simulink library "vehdynlibeom_CAVE"  (R2019b)
settings: Solver=VariableStepAuto  StartTime=0.0  StopTime=10.0  RelTol=1e-3
libraries: autolibshared x7, autolibsharedcommon x7, shared6dof_CAVE x1, autolibutils x1, sharedutil x1
Description:
  | Vehicle Dynamics Blockset: Equations of Motion
settings Model: ModifiedByFormat=The MathWorks, Inc.  Creator=The MathWorks, Inc.  LastModifiedBy=The MathWorks, Inc.
settings DataIOCC: ReturnWorkspaceOutputs=off
settings DebuggingCC: PregeneratedLibrarySubsystemCodeDiagnostic=none  ArithmeticOperatorsInVariantConditions=warning
settings SFSimCC: SimUseLocalCustomCode=off
settings RTWCC: RTWUseLocalCustomCode=off
settings CodeAppCC: StateflowObjectComments=on

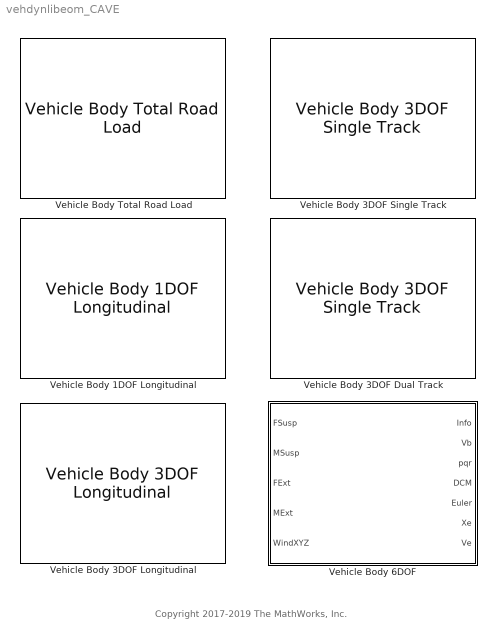
== system vehdynlibeom_CAVE ==
  note: Copyright 2017-2019 The MathWorks, Inc.
  Vehicle Body 1DOF Longitudinal : autolibshared/Vehicle Body 1DOF Longitudinal  VariantControl=SL  extFMode=off  extMMode=off  extTamb=off  wind3D=off  aMode=2  NF=2  NR=2  m=1500  a=1.4  b=1.8  h=.35  Cd=.3  Cl=0  Cpm=0  Af=4  x_o=0  xdot_o=0  Pabs=101325  T=273  g=9.81
      settings: SourceProductName=Powertrain Blockset  SourceProductBaseCode=PW
  Vehicle Body 3DOF Dual Track : autolibshared/Vehicle Body 3DOF Single Track  trackMode=Dual  inputMode=External longitudinal velocity  frontSteerMode=on  rearSteerMode=off  windMode=off  muMode=off  extFMode=off  extMMode=off  extXo=off  extpsio=off  extxdoto=off  extro=off  extYo=off  extTamb=off  extydoto=off  aMode=2  NF=2  NR=2  m=2000  a=1.4  b=1.6  h=0.35  X_o=0  xdot_o=0  CalphaMode=off  sigmaMode=on  d=0  w=[1.4,1.4]  Cy_f=12e3  Cy_r=11e3  sigma_f=.1  sigma_r=.1  alpha_f_brk=[-.1 .1]  Cy_f_data=[-9e3 9e3]  alpha_r_brk=[-.1 .1]  Cy_r_data=[-9e3 9e3]  Y_o=0  ydot_o=0  Izz=4000  psi_o=0  r_o=0  Af=2  Cd=.3  Cl=.1  Cpm=.1  beta_w=[0:0.01:0.3]  Cs=[0:0.03:0.9]  Cym=[0:0.01:0.3]  Pabs=101325  Tair=273  g=9.81  mu=1  xdot_tol=.01  Fznom=5000  Fxtire_sat=7e4  Fytire_sat=7e4  longOff=0  latOff=0  vertOff=0  wrapAng=off
      settings: SourceProductName=Powertrain Blockset  SourceProductBaseCode=PW
  Vehicle Body 3DOF Longitudinal : autolibshared/Vehicle Body 3DOF Longitudinal  VariantControl=SL  groundType=Grade angle  aMode=2  extFMode=off  extMMode=off  extTamb=off  NF=2  NR=2  m=1200  a=1.4  b=1.8  h=.35  Cd=.3  Af=2  x_o=0  xdot_o=0  Cl=.1  z_o=-.35  zdot_o=0  Iyy=3500  Cpm=.1  theta_o=0  q_o=0  FskF=[-50, -1, 0, 2, 3, 52].*1.5e4  dzsF=[-5e-3, -1e-4, 0, .2, .2001, .2051]  FsbF=[-10000 -100 -10 0 10 100 10000]  dzdotsF=[-10 -1 -.1 0 .1 1 10]  FskR=[-50, -1, 0, 2, 3, 52].*1e4  dzsR=[-5e-3, -1e-4, 0, .2, .2001, .2051]  FsbR=[-10000 -100 -10 0 10 100 10000]  dzdotsR=[-10 -1 -.1 0 .1 1 10]  Pabs=101325  T=273  g=9.81  blkID=0
      settings: SourceProductName=Powertrain Blockset  SourceProductBaseCode=PW
  Vehicle Body 3DOF Single Track : autolibshared/Vehicle Body 3DOF Single Track  trackMode=Single (bicycle)  inputMode=External longitudinal velocity  frontSteerMode=on  rearSteerMode=off  windMode=off  muMode=off  extFMode=off  extMMode=off  extXo=off  extpsio=off  extxdoto=off  extro=off  extYo=off  extTamb=off  extydoto=off  aMode=2  NF=2  NR=2  m=2000  a=1.4  b=1.6  h=0.35  X_o=0  xdot_o=0  CalphaMode=off  sigmaMode=on  d=0  w=[1.4,1.4]  Cy_f=12e3  Cy_r=11e3  sigma_f=.1  sigma_r=.1  alpha_f_brk=[-.1 .1]  Cy_f_data=[-9e3 9e3]  alpha_r_brk=[-.1 .1]  Cy_r_data=[-9e3 9e3]  Y_o=0  ydot_o=0  Izz=4000  psi_o=0  r_o=0  Af=2  Cd=.3  Cl=.1  Cpm=.1  beta_w=[0:0.01:0.3]  Cs=[0:0.03:0.9]  Cym=[0:0.01:0.3]  Pabs=101325  Tair=273  g=9.81  mu=1  xdot_tol=.01  Fznom=5000  Fxtire_sat=7e4  Fytire_sat=7e4  longOff=0  latOff=0  vertOff=0  wrapAng=off
      settings: SourceProductName=Powertrain Blockset  SourceProductBaseCode=PW
  Vehicle Body 6DOF : Subsystem  mask(Vehicle Body 6DOF 2 Axle){extPos=on, extVel=on, extEuler=on, extRotRate=on, m=2000, a=1.4, b=1.6, d=0, h=0.35, Xe_o=[0,0,0], xbdot_o=[0,0,0], eul_o=[0,0,0], p_o=[0,0,0], Iveh=[430 0 0; 0 1900 0; 0 0 2100], w=[1.9,1.9], z1m=0, z1R=[-.25,.125,.15], z1I=[1.4,-.2,.1;-.2,1.4,.1;.1,.1,2.25].*0, z2m=0, z2R=[1.4,0,.8], z2I=[1.4,-.2,.1;-.2,1.4,.1;.1,.1,2.25].*0, z3m=0, z3R=[.75,-.5,.4], z3I=[5,-.1,-2;-2,9,.1;-.1,.1,6].*0, z4m=0, z4R=[.75,.5,.4], z4I=[5,-.1,-2;-2,9,.1;-.1,.1,6].*0, z5m=0, z5R=[1.25,-.5,.4], z5I=[5,-.1,-2;-2,9,.1;-.1,.1,6].*0, z6m=0, z6R=[1.25,-.5,.4], z6I=[5,-.1,-2;-2,9,.1;-.1,.1,6].*0, z7m=0, z7R=[2,0,.25], z7I=[1.4,-.2,.1;-.2,1.4,.1;.1,.1,2.25].*0, Af=2, Cd=.3, Cl=.1, Cpm=.1, beta_w=[0:0.001:0.01], Cs=[0:0.01:0.1], Cym=[0:0.001:0.01], Pabs=101325, extTamb=off, Tair=273, g=9.81, xdot_tol=.1, longOff=0, latOff=0, vertOff=0, wrapAng=on, aMode=2}
      mask prompts: extPos "Position vector"; extVel "Velocity vector"; extEuler "Orientation vector"; extRotRate "Rotation rate vector"; m "vdynblks:vehdynVehBody6Dof:blkPrm_m"; a "vdynblks:vehdynVehBody6Dof:blkPrm_a"; b "vdynblks:vehdynVehBody6Dof:blkPrm_b"; d "vdynblks:vehdynVehBody6Dof:blkPrm_d"; h "vdynblks:vehdynVehBody6Dof:blkPrm_h"; Xe_o "vdynblks:vehdynVehBody6Dof:blkPrm_Xe_o"; xbdot_o "vdynblks:vehdynVehBody6Dof:blkPrm_xbdot_o"; eul_o "vdynblks:vehdynVehBody6Dof:blkPrm_eul_o"; p_o "vdynblks:vehdynVehBody6Dof:blkPrm_p_o"; Iveh "vdynblks:vehdynVehBody6Dof:blkPrm_Iveh"; w "vdynblks:vehdynVehBody6Dof:blkPrm_w"; z1m "vdynblks:vehdynVehBody6Dof:blkPrm_z1m"; z1R "vdynblks:vehdynVehBody6Dof:blkPrm_z1R"; z1I "vdynblks:vehdynVehBody6Dof:blkPrm_z1I"; z2m "vdynblks:vehdynVehBody6Dof:blkPrm_z2m"; z2R "vdynblks:vehdynVehBody6Dof:blkPrm_z2R"; z2I "vdynblks:vehdynVehBody6Dof:blkPrm_z2I"; z3m "vdynblks:vehdynVehBody6Dof:blkPrm_z3m"; z3R "vdynblks:vehdynVehBody6Dof:blkPrm_z3R"; z3I "vdynblks:vehdynVehBody6Dof:blkPrm_z3I"; z4m "vdynblks:vehdynVehBody6Dof:blkPrm_z4m"; z4R "vdynblks:vehdynVehBody6Dof:blkPrm_z4R"; z4I "vdynblks:vehdynVehBody6Dof:blkPrm_z4I"; z5m "vdynblks:vehdynVehBody6Dof:blkPrm_z5m"; z5R "vdynblks:vehdynVehBody6Dof:blkPrm_z5R"; z5I "vdynblks:vehdynVehBody6Dof:blkPrm_z5I"; z6m "vdynblks:vehdynVehBody6Dof:blkPrm_z6m"; z6R "vdynblks:vehdynVehBody6Dof:blkPrm_z6R"; z6I "vdynblks:vehdynVehBody6Dof:blkPrm_z6I"; z7m "vdynblks:vehdynVehBody6Dof:blkPrm_z7m"; z7R "vdynblks:vehdynVehBody6Dof:blkPrm_z7R"; z7I "vdynblks:vehdynVehBody6Dof:blkPrm_z7I"; Af "vdynblks:vehdynVehBody6Dof:blkPrm_Af"; Cd "vdynblks:vehdynVehBody6Dof:blkPrm_Cd"; Cl "vdynblks:vehdynVehBody6Dof:blkPrm_Cl"; Cpm "vdynblks:vehdynVehBody6Dof:blkPrm_Cpm"; beta_w "vdynblks:vehdynVehBody6Dof:blkPrm_beta_w"; Cs "vdynblks:vehdynVehBody6Dof:blkPrm_Cs"; Cym "vdynblks:vehdynVehBody6Dof:blkPrm_Cym"; Pabs "vdynblks:vehdynVehBody6Dof:blkPrm_Pabs"; extTamb "Air temperature"; Tair "vdynblks:vehdynVehBody6Dof:blkPrm_Tair"; g "vdynblks:vehdynVehBody6Dof:blkPrm_g"; xdot_tol "vdynblks:vehdynVehBody6Dof:blkPrm_xdot_tol"; longOff "vdynblks:vehdynVehBody6Dof:blkPrm_longOff"; latOff "vdynblks:vehdynVehBody6Dof:blkPrm_latOff"; vertOff "vdynblks:vehdynVehBody6Dof:blkPrm_vertOff"; wrapAng "Wrap Euler angles, wrapAng"
      mask help: vdynblks:vehdynVehBody6Dof:blkDesc
      mask init:
      | [~] = vehdynicon('vehdynlib6dofcar',gcb,0);
      mask Help: eval('vdynblkshelp(''vb6dof'')')
      mask Callback extTamb: [~] = vehdynicon('vehdynlib6dofcar',gcb,2);
      mask DialogControl blockConfig Prompt: Block Options
      mask DialogControl extModePanel Prompt: Initial condition input signals
      mask DialogControl vehLayoutPanel Prompt: vdynblks:vehdynVehBody6Dof:blkDlg_vehLayoutPanel
      mask DialogControl LongPanel Prompt: vdynblks:vehdynVehBody6Dof:blkDlg_LongPanel
      mask DialogControl m Prompt: Vehicle mass, m [kg]:
      mask DialogControl a Prompt: Longitudinal distance from center of mass to front axle, a [m]:
      mask DialogControl b Prompt: Longitudinal distance from center of mass to rear axle, b [m]:
      mask DialogControl d Prompt: Lateral distance from geometric centerline to center of mass, d [m]:
      mask DialogControl h Prompt: Vertical distance from center of mass to axle plane, h [m]:
      mask DialogControl Xe_o Prompt: Initial position in inertial frame [Xeo,Yeo,Zeo], Xe_o [m]:
      mask DialogControl xbdot_o Prompt: Initial velocity in body axes [xdot_o,ydot_o,zdot_o], xbdot_o [m/s]:
      mask DialogControl eul_o Prompt: Initial Euler orientation [roll, pitch, yaw], eul_o [rad]:
      mask DialogControl p_o Prompt: Initial body rotation rates [p,q,r], p_o [rad/s]:
      mask DialogControl Iveh Prompt: Chassis inertia tensor, Iveh [kg*m^2]:
      mask DialogControl w Prompt: Track widths [front, rear], w [m]:
      mask DialogControl loadPanel Prompt: vdynblks:vehdynVehBody6Dof:blkDlg_loadPanel
      mask DialogControl zone1Panel Prompt: vdynblks:vehdynVehBody6Dof:blkDlg_zone1Panel
      mask DialogControl z1m Prompt: Mass, z1m [kg]:
      mask DialogControl z1R Prompt: Distance vector from front axle, z1R [m]:
      mask DialogControl z1I Prompt: Inertia tensor, z1I, [kg*m^2]:
      mask DialogControl zone2Panel Prompt: vdynblks:vehdynVehBody6Dof:blkDlg_zone2Panel
      mask DialogControl z2m Prompt: Mass, z2m [kg]:
      mask DialogControl z2R Prompt: Distance vector from front axle, z2R [m]:
      mask DialogControl z2I Prompt: Inertia tensor, z2I, [kg*m^2]:
      mask DialogControl zone3Panel Prompt: vdynblks:vehdynVehBody6Dof:blkDlg_zone3Panel
      mask DialogControl z3m Prompt: Mass, z3m [kg]:
      mask DialogControl z3R Prompt: Distance vector from front axle, z3R [m]:
      mask DialogControl z3I Prompt: Inertia tensor, z3I, [kg*m^2]:
      mask DialogControl zone4Panel Prompt: vdynblks:vehdynVehBody6Dof:blkDlg_zone4Panel
      mask DialogControl z4m Prompt: Mass, z4m [kg]:
      mask DialogControl z4R Prompt: Distance vector from front axle, z4R [m]:
      mask DialogControl z4I Prompt: Inertia tensor, z4I, [kg*m^2]:
      mask DialogControl zone5Panel Prompt: vdynblks:vehdynVehBody6Dof:blkDlg_zone5Panel
      mask DialogControl z5m Prompt: Mass, z5m [kg]:
      mask DialogControl z5R Prompt: Distance vector from front axle, z5R [m]:
      mask DialogControl z5I Prompt: Inertia tensor, z5I, [kg*m^2]:
      mask DialogControl zone6Panel Prompt: vdynblks:vehdynVehBody6Dof:blkDlg_zone6Panel
      mask DialogControl z6m Prompt: Mass, z6m [kg]:
      mask DialogControl z6R Prompt: Distance vector from front axle, z6R [m]:
      mask DialogControl z6I Prompt: Inertia tensor, z6I, [kg*m^2]:
      mask DialogControl zone7Panel Prompt: vdynblks:vehdynVehBody6Dof:blkDlg_zone7Panel
      mask DialogControl z7m Prompt: Mass, z7m [kg]:
      mask DialogControl z7R Prompt: Distance vector from front axle, z7R [m]:
      mask DialogControl z7I Prompt: Inertia tensor, z7I, [kg*m^2]:
      mask DialogControl AeroParams Prompt: vdynblks:vehdynVehBody6Dof:blkDlg_AeroParams
      mask DialogControl Af Prompt: Longitudinal drag area, Af [m^2]:
      mask DialogControl Cd Prompt: Longitudinal drag coefficient, Cd [-]:
      mask DialogControl Cl Prompt: Longitudinal lift coefficient, Cl [-]:
      mask DialogControl Cpm Prompt: Longitudinal drag pitch moment, Cpm [-]:
      mask DialogControl beta_w Prompt: Relative wind angle vector, beta_w [rad]:
      mask DialogControl Cs Prompt: Side force coefficient vector, Cs [-]:
      mask DialogControl Cym Prompt: Yaw moment coefficient vector, Cym [-]:
      mask DialogControl EnviroPanel Prompt: vdynblks:vehdynVehBody6Dof:blkDlg_EnviroPanel
      mask DialogControl Pabs Prompt: Absolute Pressure, Pabs [Pa]:
      mask DialogControl Tair Prompt: Air temperature, Tair [K]:
      mask DialogControl g Prompt: Gravitational acceleration, g [m/s^2]:
      mask DialogControl SimPanel Prompt: vdynblks:vehdynVehBody6Dof:blkDlg_SimPanel
      mask DialogControl xdot_tol Prompt: Longitudinal velocity tolerance, xdot_tol [m/s]:
      mask DialogControl longOff Prompt: Geometric longitudinal offset from axle plane, longOff [m]:
      mask DialogControl latOff Prompt: Geometric lateral offset from axle plane, latOff [m]:
      mask DialogControl vertOff Prompt: Geometric vertical offset from axle plane, vertOff [m]:
      mask Display:
      | try
      |     IconInfo = vehdynicon('vehdynlib6dofcar',gcb,8);
      | 
      |     image(IconInfo.image, IconInfo.position);
      | 
      |     for i = 1:numel(IconInfo.lconn)
      |         port_label('lconn', i, IconInfo.lconn{i})
      |     end
      | 
      |     for j = 1:numel(IconInfo.rconn)
      |         port_label('rconn', j, IconInfo.rconn{j})
      |     end
      | 
      |     for k = 1:numel(IconInfo.input)
      |         port_label('input', k, IconInfo.input{k})
      |     end
      | 
      |     for m = 1:numel(IconInfo.output)
      |         port_label('output', m, IconInfo.output{m})
      |     end
      | catch
      |     fprintf('Vehicle Body \n 6DOF Car')
      | end
  Vehicle Body Total Road Load : autolibshared/Vehicle Body Total Road Load  VariantControl=SL1dof  input_type=Force  aMode=2  m=1200  a=196  b=2.232  c=0.389  g=9.81  x_o=0  xdot_o=0
      settings: SourceProductName=Powertrain Blockset  SourceProductBaseCode=PW

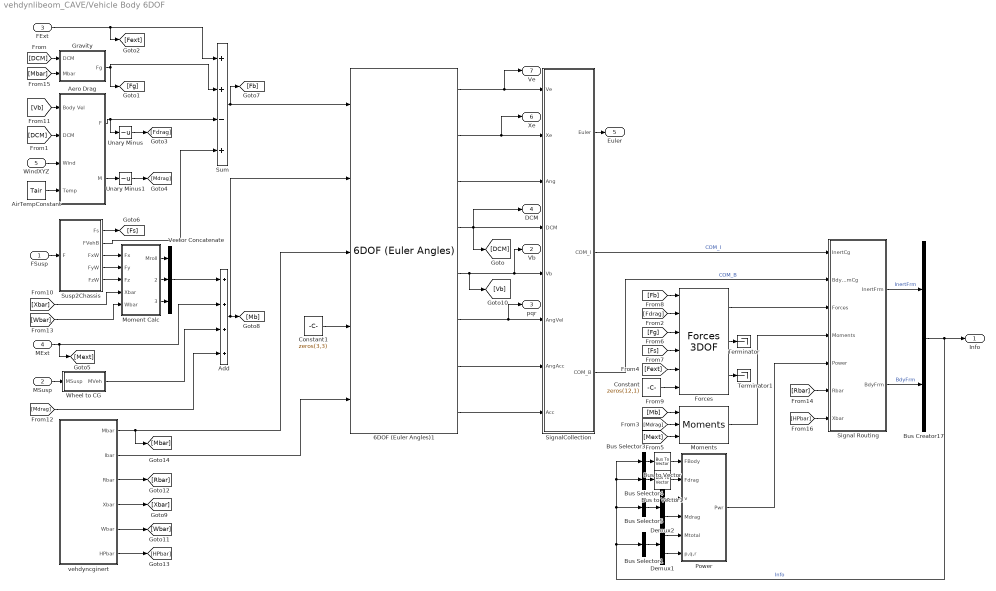
== system vehdynlibeom_CAVE/Vehicle Body 6DOF ==
  FSusp : Inport  Unit=N
  MSusp : Inport  Port=2  Unit=N*m
  FExt : Inport  Port=3  Unit=N
  MExt : Inport  Port=4  Unit=N*m
  WindXYZ : Inport  Port=5  Unit=m/s
  6DOF (Euler Angles)1 : shared6dof_CAVE/6DOF (Euler Angles)  units=Metric (MKS)  mtype=Custom Variable  rep=Euler Angles  xme_0=Xe_o  Vm_0=xbdot_o  eul_0=eul_o  pm_0=p_o  mass_0=1.0  mass_e=0.5  mass_f=2.0  inertia=eye(3)  inertia_e=eye(3)  inertia_f=2*eye(3)  k_quat=1.0  vre_flag=off  abi_flag=off  aMode=aMode  xme_statename=''  Vm_statename=''  eul_statename=''  quat_statename=''  pm_statename=''  mass_statename=''
  Add : Sum  Inputs=++++
  Aero Drag : Subsystem
  AirTempConstant : Constant  Value=Tair
  Bus Creator17 : BusCreator  Inputs=2
  Bus Selector1 : BusSelector  OutputSignals=BdyFrm.Moments.Body.Mx,BdyFrm.Moments.Body.My,BdyFrm.Moments.Body.Mz,BdyFrm.Cg.AngVel.p,BdyFrm.Cg.AngVel.q,BdyFrm.Cg.AngVel.r  OutputAsBus=on
  Bus Selector3 : BusSelector  OutputSignals=BdyFrm.Forces.Body.Fx,BdyFrm.Forces.Body.Fy,BdyFrm.Forces.Body.Fz  OutputAsBus=on
  Bus Selector4 : BusSelector  OutputSignals=BdyFrm.Forces.Drag.Fx,BdyFrm.Forces.Drag.Fy,BdyFrm.Forces.Drag.Fz  OutputAsBus=on
  Bus Selector5 : BusSelector  OutputSignals=BdyFrm.Cg.Vel.xdot,BdyFrm.Cg.Vel.ydot,BdyFrm.Cg.Vel.zdot,BdyFrm.Moments.Drag.Mx,BdyFrm.Moments.Drag.My,BdyFrm.Moments.Drag.Mz  OutputAsBus=on
  Bus to Vector : BusToVector
  Bus to Vector1 : BusToVector
  Constant : Constant  Value=zeros(12,1)
  Constant1 : Constant  Value=zeros(3,3)
  Demux1 : Demux  Outputs=[3, 3]
  Demux2 : Demux  Outputs=[3, 3]
  Forces : autolibshared/Vehicle Body 3DOF Single Track/Signal Routing/Signal Routing Dual/Forces 3DOF  SystemSampleTime=-1  VariantControl=2  Latency=0  AutoFrameSizeCalculation=off
      settings: SourceProductName=Powertrain Blockset  SourceProductBaseCode=PW
  Gravity : Subsystem
  Moment Calc : Subsystem
  Moments : autolibsharedcommon/Bus Creation/Moments  SystemSampleTime=-1  Latency=0  AutoFrameSizeCalculation=off
      settings: SourceProductName=Powertrain Blockset  SourceProductBaseCode=PW
  Power : Subsystem  VariantControl=2
  Signal Routing : Subsystem  VariantControl=2
  SignalCollection : Subsystem
  Sum : Sum  Inputs=++-+  SaturateOnIntegerOverflow=on  InputSameDT=on  OutDataTypeStr=Inherit: Same as first input
  Susp2Chassis : Subsystem
  Terminator : Terminator
  Terminator1 : Terminator
  Unary Minus : UnaryMinus
  Unary Minus1 : UnaryMinus
  Vector Concatenate : Concatenate  NumInputs=3
  Wheel to CG : Subsystem
  vehdyncginert : MATLAB Function  TreatAsAtomicUnit=on
  Info : Outport  VectorParamsAs1DForOutWhenUnconnected=off
  Vb : Outport  Port=2  Unit=m/s  VectorParamsAs1DForOutWhenUnconnected=off
  pqr : Outport  Port=3  Unit=rad/s  VectorParamsAs1DForOutWhenUnconnected=off
  DCM : Outport  Port=4  VectorParamsAs1DForOutWhenUnconnected=off
  Euler : Outport  Port=5  Unit=rad  VectorParamsAs1DForOutWhenUnconnected=off
  Xe : Outport  Port=6  Unit=m  VectorParamsAs1DForOutWhenUnconnected=off
  Ve : Outport  Port=7  Unit=m/s  VectorParamsAs1DForOutWhenUnconnected=off
  wires:
  Vector Concatenate/1 -> Add/1
  Susp2Chassis/1(Fs) -> [Fs]
  Moment Calc/3(Myaw) -> Vector Concatenate/3
  Moment Calc/1(Mroll) -> Vector Concatenate/1
  Moment Calc/2(Mpitch) -> Vector Concatenate/2
  MSusp/1 -> Wheel to CG/1(MSusp)
  FSusp/1 -> Susp2Chassis/1(F)
  Gravity/1(Fg) -> Sum/2, [Fg]
  6DOF (Euler Angles)1/7 -> SignalCollection/7(AngAcc)
  [DCM] -> Gravity/1(DCM)
  WindXYZ/1 -> Aero Drag/3(Wind)
  [Vb] -> Aero Drag/1(Body Vel)
  Add/1 -> 6DOF (Euler Angles)1/2, [Mb]
  6DOF (Euler Angles)1/4 -> [DCM], SignalCollection/4(DCM), DCM/1
  Aero Drag/2(M) -> Unary Minus1/1
  Aero Drag/1(F) -> Sum/3, Unary Minus/1
  [DCM] -> Aero Drag/2(DCM)
  Sum/1 -> 6DOF (Euler Angles)1/1, [Fb]
  6DOF (Euler Angles)1/8 -> SignalCollection/8(Acc)
  FExt/1 -> Sum/1, [Fext]
  Bus Selector1/1 -> Demux1/1
  Bus Selector3/1 -> Bus to Vector/1
  Bus Selector5/1 -> Demux2/1
  Bus Selector4/1 -> Bus to Vector1/1
  Bus Creator17/1 -> Bus Selector3/1, Bus Selector4/1, Bus Selector5/1, Bus Selector1/1, Info/1  "Info"
  Demux1/2 -> Power/6(p,q,r)
  Signal Routing/1(InertFrm) -> Bus Creator17/1  "InertFrm"
  Demux1/1 -> Power/5(Mtotal)
  Power/1(Pwr) -> Signal Routing/5(Power)
  Signal Routing/2(BdyFrm) -> Bus Creator17/2  "BdyFrm"
  SignalCollection/2(COM_I) -> Signal Routing/1(InertCg)  "COM_I"
  SignalCollection/3(COM_B) -> Signal Routing/2(BdyFrmCg)  "COM_B"
  Forces/1 -> Signal Routing/3(Forces)
  Moments/1 -> Signal Routing/4(Moments)
  [Fdrag] -> Forces/2
  [Mdrag] -> Moments/2
  [Fext] -> Forces/5
  [Mext] -> Moments/3
  [Fg] -> Forces/3
  [Fb] -> Forces/1
  [Mb] -> Moments/1
  Constant/1 -> Forces/6
  Forces/2 -> Terminator/1
  Forces/3 -> Terminator1/1
  Susp2Chassis/2(FVehB) -> Sum/4
  MExt/1 -> Add/2, [Mext]
  Wheel to CG/1(MVeh) -> Add/3
  [Fs] -> Forces/4
  Susp2Chassis/3(FxW) -> Moment Calc/1(Fx)
  Susp2Chassis/4(FyW) -> Moment Calc/2(Fy)
  Susp2Chassis/5(FzW) -> Moment Calc/3(Fz)
  6DOF (Euler Angles)1/3 -> SignalCollection/3(Ang)
  6DOF (Euler Angles)1/5 -> [Vb], Vb/1, SignalCollection/5(Vb)
  6DOF (Euler Angles)1/6 -> pqr/1, SignalCollection/6(AngVel)
  6DOF (Euler Angles)1/1 -> Ve/1, SignalCollection/1(Ve)
  6DOF (Euler Angles)1/2 -> Xe/1, SignalCollection/2(Xe)
  [Mdrag] -> Add/4
  vehdyncginert/1(Mbar) -> 6DOF (Euler Angles)1/3, [Mbar]
  vehdyncginert/3(Rbar) -> [Rbar]
  Constant1/1 -> 6DOF (Euler Angles)1/4
  vehdyncginert/2(Ibar) -> 6DOF (Euler Angles)1/5
  [Xbar] -> Moment Calc/4(Xbar)
  vehdyncginert/4(Xbar) -> [Xbar]
  vehdyncginert/5(Wbar) -> [Wbar]
  [Wbar] -> Moment Calc/5(Wbar)
  [HPbar] -> Signal Routing/7(Xbar)
  vehdyncginert/6(HPbar) -> [HPbar]
  [Rbar] -> Signal Routing/6(Rbar)
  Bus to Vector/1 -> Power/1(FBody)
  Bus to Vector1/1 -> Power/2(Fdrag)
  Demux2/1 -> Power/3(v)
  Demux2/2 -> Power/4(Mdrag)
  AirTempConstant/1 -> Aero Drag/4(Temp)
  SignalCollection/1(Euler) -> Euler/1
  [Mbar] -> Gravity/2(Mbar)
  Unary Minus/1 -> [Fdrag]
  Unary Minus1/1 -> [Mdrag]

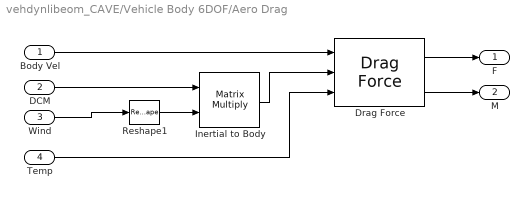
== system vehdynlibeom_CAVE/Vehicle Body 6DOF/Aero Drag ==
  Body Vel : Inport
  DCM : Inport  Port=2
  Wind : Inport  Port=3
  Temp : Inport  Port=4  Unit=K
  Drag Force : autolibsharedcommon/Vehicle Body 3dof/Drag Force  A=Af  beta_w=beta_w  Cd=Cd  Cs=Cs  Cl=Cl  Cpm=Cpm  Lcpm=a+b  Crm=beta_w.*eps  Cym=Cym  R=287.058  Pabs=Pabs
      settings: SourceProductName=Powertrain Blockset  SourceProductBaseCode=PW
  Inertial to Body : Product  Multiplication=Matrix(*)  SaturateOnIntegerOverflow=on  InputSameDT=on  OutDataTypeStr=Inherit: Same as first input
  Reshape1 : Reshape
  F : Outport  VectorParamsAs1DForOutWhenUnconnected=off
  M : Outport  Port=2  VectorParamsAs1DForOutWhenUnconnected=off
  wires:
  Body Vel/1 -> Drag Force/1
  Inertial to Body/1 -> Drag Force/2
  Drag Force/1 -> F/1
  Drag Force/2 -> M/1
  Reshape1/1 -> Inertial to Body/2
  DCM/1 -> Inertial to Body/1
  Wind/1 -> Reshape1/1
  Temp/1 -> Drag Force/3

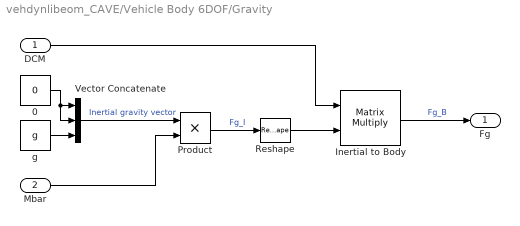
== system vehdynlibeom_CAVE/Vehicle Body 6DOF/Gravity ==
  DCM : Inport
  Mbar : Inport  Port=2
  0 : Constant  Value=0
  Inertial to Body : Product  Multiplication=Matrix(*)  SaturateOnIntegerOverflow=on  InputSameDT=on  OutDataTypeStr=Inherit: Same as first input
  Product : Product
  Reshape : Reshape
  Vector Concatenate : Concatenate  NumInputs=3
  g : Constant  Value=g
  Fg : Outport  VectorParamsAs1DForOutWhenUnconnected=off
  wires:
  DCM/1 -> Inertial to Body/1
  Product/1 -> Reshape/1  "Fg_I"
  Reshape/1 -> Inertial to Body/2
  g/1 -> Vector Concatenate/3
  Inertial to Body/1 -> Fg/1  "Fg_B"
  Mbar/1 -> Product/2
  Vector Concatenate/1 -> Product/1  "Inertial gravity vector"
  0/1 -> Vector Concatenate/2, Vector Concatenate/1

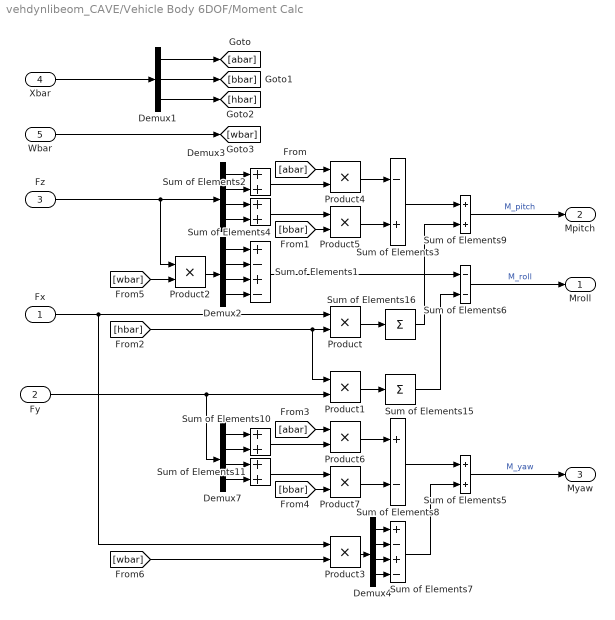
== system vehdynlibeom_CAVE/Vehicle Body 6DOF/Moment Calc ==
  Fx : Inport
  Fy : Inport  Port=2
  Fz : Inport  Port=3
  Xbar : Inport  Port=4
  Wbar : Inport  Port=5
  Demux1 : Demux  Outputs=3
  Demux{2..4,7} (4 alike) : Demux
  Product{,1..7} (8 alike) : Product
  Sum of Elements1 : Sum  Inputs=+-+-
  Sum of Elements{2,4..5,9..11} (6 alike) : Sum
  Sum of Elements15 : Sum  Inputs=+
  Sum of Elements16 : Sum  Inputs=+
  Sum of Elements3 : Sum  Inputs=-+
  Sum of Elements6 : Sum  Inputs=--
  Sum of Elements7 : Sum  Inputs=+-+-
  Sum of Elements8 : Sum  Inputs=+-
  Mroll : Outport  VectorParamsAs1DForOutWhenUnconnected=off
  Mpitch : Outport  Port=2  VectorParamsAs1DForOutWhenUnconnected=off
  Myaw : Outport  Port=3  VectorParamsAs1DForOutWhenUnconnected=off
  wires:
  Product1/1 -> Sum of Elements15/1
  Product/1 -> Sum of Elements16/1
  Sum of Elements6/1 -> Mroll/1  "M_roll"
  Sum of Elements9/1 -> Mpitch/1  "M_pitch"
  Product4/1 -> Sum of Elements3/1
  Demux2/1 -> Sum of Elements1/1
  Sum of Elements7/1 -> Sum of Elements5/2
  Product5/1 -> Sum of Elements3/2
  Sum of Elements16/1 -> Sum of Elements9/2
  Sum of Elements5/1 -> Myaw/1  "M_yaw"
  Sum of Elements8/1 -> Sum of Elements5/1
  Sum of Elements15/1 -> Sum of Elements6/2
  Demux3/2 -> Sum of Elements2/2
  Demux3/1 -> Sum of Elements2/1
  Demux3/4 -> Sum of Elements4/2
  [hbar] -> Product1/1, Product/2
  Sum of Elements3/1 -> Sum of Elements9/1
  Demux3/3 -> Sum of Elements4/1
  Sum of Elements4/1 -> Product5/1
  Sum of Elements2/1 -> Product4/2
  Sum of Elements1/1 -> Sum of Elements6/1
  Fz/1 -> Product2/1, Demux3/1
  Fx/1 -> Product3/1, Product/1
  Demux2/4 -> Sum of Elements1/4
  Demux4/4 -> Sum of Elements7/4
  Demux4/1 -> Sum of Elements7/1
  Fy/1 -> Demux7/1, Product1/2
  Demux2/2 -> Sum of Elements1/2
  Demux2/3 -> Sum of Elements1/3
  Product2/1 -> Demux2/1
  Demux4/2 -> Sum of Elements7/2
  Demux4/3 -> Sum of Elements7/3
  Product3/1 -> Demux4/1
  [wbar] -> Product3/2
  [abar] -> Product4/1
  [bbar] -> Product5/2
  [bbar] -> Product7/2
  [abar] -> Product6/1
  Sum of Elements10/1 -> Product6/2
  Sum of Elements11/1 -> Product7/1
  Product7/1 -> Sum of Elements8/2
  Product6/1 -> Sum of Elements8/1
  Demux7/3 -> Sum of Elements11/1
  Demux7/4 -> Sum of Elements11/2
  Demux7/1 -> Sum of Elements10/1
  Demux7/2 -> Sum of Elements10/2
  Demux1/3 -> [hbar]
  Xbar/1 -> Demux1/1
  [wbar] -> Product2/2
  Demux1/2 -> [bbar]
  Demux1/1 -> [abar]
  Wbar/1 -> [wbar]

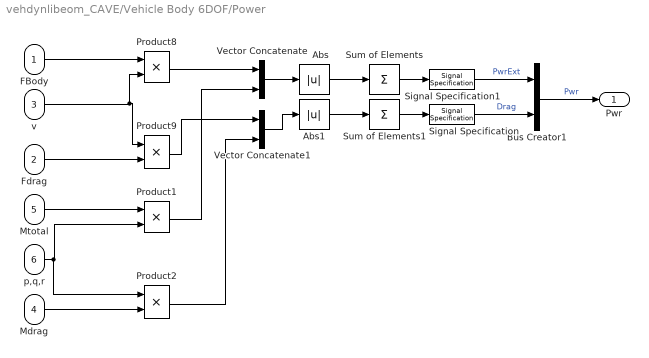
== system vehdynlibeom_CAVE/Vehicle Body 6DOF/Power ==
  FBody : Inport
  Fdrag : Inport  Port=2
  v : Inport  Port=3
  Mdrag : Inport  Port=4
  Mtotal : Inport  Port=5
  p,q,r : Inport  Port=6
  Abs : Abs  ZeroCross=off
  Abs1 : Abs  ZeroCross=off
  Bus Creator1 : BusCreator  Inputs=2
  Product{1..2,8..9} (4 alike) : Product
  Signal Specification : SignalSpecification  Unit=W
  Signal Specification1 : SignalSpecification  Unit=W
  Sum of Elements : Sum  Inputs=+
  Sum of Elements1 : Sum  Inputs=+
  Vector Concatenate : Concatenate
  Vector Concatenate1 : Concatenate
  Pwr : Outport  VectorParamsAs1DForOutWhenUnconnected=off
  wires:
  Bus Creator1/1 -> Pwr/1  "Pwr"
  Product9/1 -> Vector Concatenate1/1
  Signal Specification1/1 -> Bus Creator1/1  "PwrExt"
  Signal Specification/1 -> Bus Creator1/2  "Drag"
  Product8/1 -> Vector Concatenate/1
  Fdrag/1 -> Product9/2
  FBody/1 -> Product8/1
  Abs/1 -> Sum of Elements/1
  Abs1/1 -> Sum of Elements1/1
  Sum of Elements/1 -> Signal Specification1/1
  Sum of Elements1/1 -> Signal Specification/1
  Mtotal/1 -> Product1/1
  Mdrag/1 -> Product2/2
  Product1/1 -> Vector Concatenate/2
  Product2/1 -> Vector Concatenate1/2
  p,q,r/1 -> Product2/1, Product1/2
  Vector Concatenate/1 -> Abs/1
  Vector Concatenate1/1 -> Abs1/1
  v/1 -> Product9/1, Product8/2

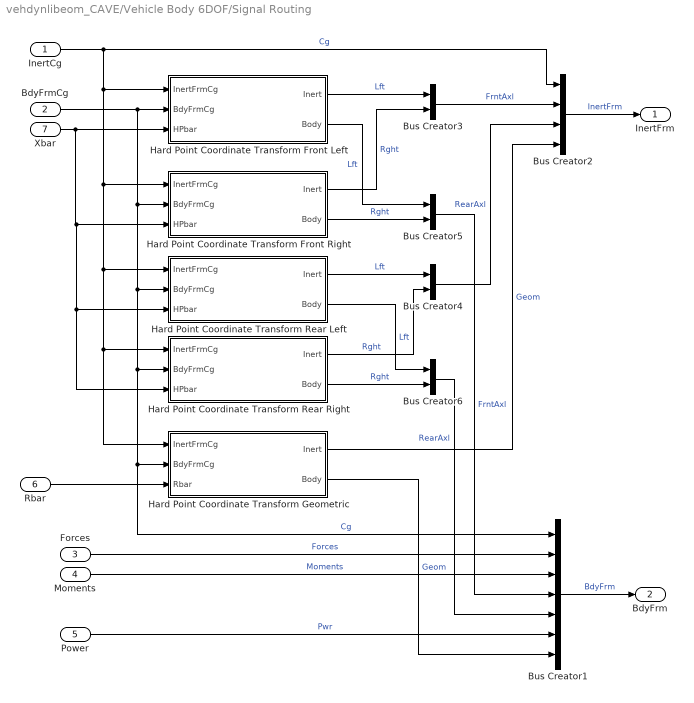
== system vehdynlibeom_CAVE/Vehicle Body 6DOF/Signal Routing ==
  InertCg : Inport
  BdyFrmCg : Inport  Port=2
  Forces : Inport  Port=3
  Moments : Inport  Port=4
  Power : Inport  Port=5
  Rbar : Inport  Port=6
  Xbar : Inport  Port=7
  Bus Creator1 : BusCreator  Inputs=7
  Bus Creator2 : BusCreator  Inputs=4
  Bus Creator{3..6} (4 alike) : BusCreator  Inputs=2
  Hard Point Coordinate Transform Front Left : Subsystem
  Hard Point Coordinate Transform Front Right : Subsystem
  Hard Point Coordinate Transform Geometric : Subsystem
  Hard Point Coordinate Transform Rear Left : Subsystem
  Hard Point Coordinate Transform Rear Right : Subsystem
  InertFrm : Outport  VectorParamsAs1DForOutWhenUnconnected=off
  BdyFrm : Outport  Port=2  VectorParamsAs1DForOutWhenUnconnected=off
  wires:
  Hard Point Coordinate Transform Geometric/1(Inert) -> Bus Creator2/4  "Geom"
  Hard Point Coordinate Transform Geometric/2(Body) -> Bus Creator1/7  "Geom"
  Power/1 -> Bus Creator1/6  "Pwr"
  Forces/1 -> Bus Creator1/2  "Forces"
  BdyFrmCg/1 -> Hard Point Coordinate Transform Geometric/2(BdyFrmCg), Bus Creator1/1, Hard Point Coordinate Transform Rear Right/2(BdyFrmCg), Hard Point Coordinate Transform Rear Left/2(BdyFrmCg), Hard Point Coordinate Transform Front Right/2(BdyFrmCg), Hard Point Coordinate Transform Front Left/2(BdyFrmCg)  "Cg"
  Bus Creator3/1 -> Bus Creator2/2  "FrntAxl"
  Bus Creator1/1 -> BdyFrm/1  "BdyFrm"
  Bus Creator2/1 -> InertFrm/1  "InertFrm"
  Bus Creator4/1 -> Bus Creator2/3  "RearAxl"
  InertCg/1 -> Hard Point Coordinate Transform Rear Left/1(InertFrmCg), Hard Point Coordinate Transform Rear Right/1(InertFrmCg), Hard Point Coordinate Transform Geometric/1(InertFrmCg), Hard Point Coordinate Transform Front Right/1(InertFrmCg), Hard Point Coordinate Transform Front Left/1(InertFrmCg), Bus Creator2/1  "Cg"
  Bus Creator5/1 -> Bus Creator1/4  "FrntAxl"
  Moments/1 -> Bus Creator1/3  "Moments"
  Hard Point Coordinate Transform Front Left/1(Inert) -> Bus Creator3/1  "Lft"
  Hard Point Coordinate Transform Front Right/1(Inert) -> Bus Creator3/2  "Rght"
  Hard Point Coordinate Transform Rear Left/1(Inert) -> Bus Creator4/1  "Lft"
  Hard Point Coordinate Transform Rear Right/1(Inert) -> Bus Creator4/2  "Rght"
  Hard Point Coordinate Transform Rear Right/2(Body) -> Bus Creator6/2  "Rght"
  Hard Point Coordinate Transform Rear Left/2(Body) -> Bus Creator6/1  "Lft"
  Hard Point Coordinate Transform Front Right/2(Body) -> Bus Creator5/2  "Rght"
  Hard Point Coordinate Transform Front Left/2(Body) -> Bus Creator5/1  "Lft"
  Bus Creator6/1 -> Bus Creator1/5  "RearAxl"
  Xbar/1 -> Hard Point Coordinate Transform Front Right/3(HPbar), Hard Point Coordinate Transform Rear Right/3(HPbar), Hard Point Coordinate Transform Rear Left/3(HPbar), Hard Point Coordinate Transform Front Left/3(HPbar)
  Rbar/1 -> Hard Point Coordinate Transform Geometric/3(Rbar)

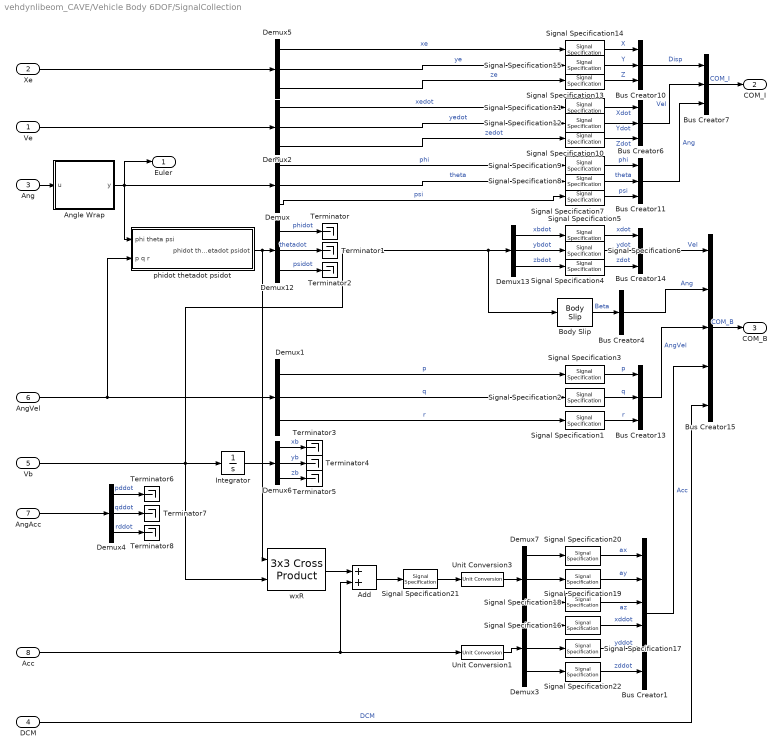
== system vehdynlibeom_CAVE/Vehicle Body 6DOF/SignalCollection ==
  Ve : Inport
  Xe : Inport  Port=2
  Ang : Inport  Port=3
  DCM : Inport  Port=4
  Vb : Inport  Port=5
  AngVel : Inport  Port=6
  AngAcc : Inport  Port=7
  Acc : Inport  Port=8
  Add : Sum
  Angle Wrap : Subsystem  VariantControlMode=Label  Variant=on  VariantControl=Variant1  LabelModeActiveChoice=None
  Body Slip : autolibshared/Vehicle Body 3DOF Single Track/Signal Routing/Signal Routing/state2bus/Body Slip  mask{xdot_tol=xdot_tol}
      mask prompts: xdot_tol "Longituindal low speed tolerance, xdot_tol [m/s]:"
      settings: SourceProductName=Powertrain Blockset  SourceProductBaseCode=PW
  Bus Creator1 : BusCreator  Inputs=6
  Bus Creator{6..7,10..11,13..14} (6 alike) : BusCreator  Inputs=3
  Bus Creator15 : BusCreator  Inputs=5
  Bus Creator4 : BusCreator  Inputs=1
  Demux{,1..7,12..13} (10 alike) : Demux  Outputs=3
  Integrator : Integrator  InitialCondition=[0 0 0]
  Signal Specification1 : SignalSpecification  Unit=rad/s
  Signal Specification{4..6,10..12} (6 alike) : SignalSpecification  Unit=m/s
  Signal Specification13 : SignalSpecification  Unit=m
  Signal Specification14 : SignalSpecification  Unit=m
  Signal Specification15 : SignalSpecification  Unit=m
  Signal Specification{16..17,21..22} (4 alike) : SignalSpecification  Unit=m/s^2
  Signal Specification18 : SignalSpecification  Unit=gn
  Signal Specification19 : SignalSpecification  Unit=gn
  Signal Specification2 : SignalSpecification  Unit=rad/s
  Signal Specification20 : SignalSpecification  Unit=gn
  Signal Specification3 : SignalSpecification  Unit=rad/s
  Signal Specification7 : SignalSpecification  Unit=rad
  Signal Specification8 : SignalSpecification  Unit=rad
  Signal Specification9 : SignalSpecification  Unit=rad
  Terminator{,1..8} (9 alike) : Terminator
  Unit Conversion1 : UnitConversion
  Unit Conversion3 : UnitConversion
  phidot thetadot psidot : Subsystem
  wxR : sharedutil/3x3 Cross Product  aMode=aMode
      settings: SourceProductBaseCode=AE
  Euler : Outport  Unit=rad  VectorParamsAs1DForOutWhenUnconnected=off
  COM_I : Outport  Port=2  VectorParamsAs1DForOutWhenUnconnected=off
  COM_B : Outport  Port=3  VectorParamsAs1DForOutWhenUnconnected=off
  wires:
  AngAcc/1 -> Demux4/1
  Demux/1 -> Signal Specification9/1  "phi"
  Demux/2 -> Signal Specification8/1  "theta"
  Demux/3 -> Signal Specification7/1  "psi"
  Demux1/2 -> Signal Specification2/1  "q"
  Demux1/3 -> Signal Specification1/1  "r"
  Demux2/1 -> Signal Specification11/1  "xedot"
  Demux2/2 -> Signal Specification12/1  "yedot"
  Demux2/3 -> Signal Specification10/1  "zedot"
  Demux3/1 -> Signal Specification16/1
  Demux3/2 -> Signal Specification17/1
  Demux3/3 -> Signal Specification22/1
  Xe/1 -> Demux5/1
  Demux5/1 -> Signal Specification14/1  "xe"
  Demux5/2 -> Signal Specification15/1  "ye"
  Demux5/3 -> Signal Specification13/1  "ze"
  Demux4/1 -> Terminator6/1  "pddot"
  Demux4/2 -> Terminator7/1  "qddot"
  Demux4/3 -> Terminator8/1  "rddot"
  Ang/1 -> Angle Wrap/1("u ")
  Demux12/1 -> Terminator/1  "phidot"
  Demux12/2 -> Terminator1/1  "thetadot"
  Demux12/3 -> Terminator2/1  "psidot"
  phidot thetadot psidot/1(phidot thetadot psidot) -> wxR/1, Demux12/1
  AngVel/1 -> phidot thetadot psidot/2(p q r), Demux1/1
  Demux13/1 -> Signal Specification5/1  "xbdot"
  Demux13/2 -> Signal Specification6/1  "ybdot"
  Demux13/3 -> Signal Specification4/1  "zbdot"
  Vb/1 -> wxR/2, Body Slip/1, Demux13/1, Integrator/1
  Bus Creator7/1 -> COM_I/1  "COM_I"
  Demux1/1 -> Signal Specification3/1  "p"
  Integrator/1 -> Demux6/1
  Demux6/1 -> Terminator3/1  "xb"
  Demux6/2 -> Terminator4/1  "yb"
  Demux6/3 -> Terminator5/1  "zb"
  Signal Specification9/1 -> Bus Creator11/1  "phi"
  Bus Creator13/1 -> Bus Creator15/3  "AngVel"
  Signal Specification3/1 -> Bus Creator13/1  "p"
  Signal Specification1/1 -> Bus Creator13/3  "r"
  Signal Specification6/1 -> Bus Creator14/2  "ydot"
  Signal Specification7/1 -> Bus Creator11/3  "psi"
  Bus Creator11/1 -> Bus Creator7/3  "Ang"
  Signal Specification4/1 -> Bus Creator14/3  "zdot"
  Bus Creator6/1 -> Bus Creator7/2  "Vel"
  Signal Specification8/1 -> Bus Creator11/2  "theta"
  Bus Creator15/1 -> COM_B/1  "COM_B"
  Signal Specification11/1 -> Bus Creator6/1  "Xdot"
  Signal Specification5/1 -> Bus Creator14/1  "xdot"
  Signal Specification13/1 -> Bus Creator10/3  "Z"
  Signal Specification2/1 -> Bus Creator13/2  "q"
  Signal Specification12/1 -> Bus Creator6/2  "Ydot"
  Signal Specification10/1 -> Bus Creator6/3  "Zdot"
  Bus Creator14/1 -> Bus Creator15/1  "Vel"
  Signal Specification15/1 -> Bus Creator10/2  "Y"
  Signal Specification14/1 -> Bus Creator10/1  "X"
  Bus Creator10/1 -> Bus Creator7/1  "Disp"
  Bus Creator1/1 -> Bus Creator15/4  "Acc"
  Signal Specification18/1 -> Bus Creator1/3  "az"
  Signal Specification20/1 -> Bus Creator1/1  "ax"
  Signal Specification19/1 -> Bus Creator1/2  "ay"
  wxR/1 -> Add/1
  Demux7/2 -> Signal Specification19/1
  Demux7/1 -> Signal Specification20/1
  Demux7/3 -> Signal Specification18/1
  Acc/1 -> Add/2, Unit Conversion1/1
  Add/1 -> Signal Specification21/1
  Unit Conversion3/1 -> Demux7/1
  Signal Specification21/1 -> Unit Conversion3/1
  Unit Conversion1/1 -> Demux3/1
  Signal Specification17/1 -> Bus Creator1/5  "yddot"
  Signal Specification22/1 -> Bus Creator1/6  "zddot"
  Signal Specification16/1 -> Bus Creator1/4  "xddot"
  DCM/1 -> Bus Creator15/5  "DCM"
  Bus Creator4/1 -> Bus Creator15/2  "Ang"
  Body Slip/1 -> Bus Creator4/1  "Beta"
  Ve/1 -> Demux2/1
  Angle Wrap/1(" y") -> Euler/1, Demux/1, phidot thetadot psidot/1(phi theta psi)

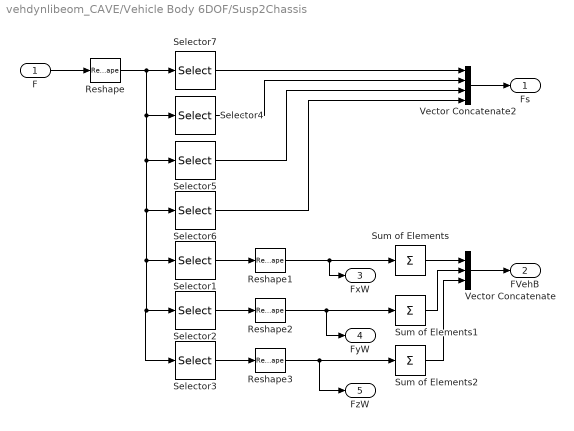
== system vehdynlibeom_CAVE/Vehicle Body 6DOF/Susp2Chassis ==
  F : Inport
  Reshape : Reshape  OutputDimensionality=Customize  OutputDimensions=[3,4]
  Reshape1 : Reshape
  Reshape2 : Reshape
  Reshape3 : Reshape
  Selector1 : Selector  NumberOfDimensions=2  InputPortWidth=3  IndexOptions=Index vector (dialog),Select all  Indices=[1],1  OutputSizes=1,1
  Selector2 : Selector  NumberOfDimensions=2  InputPortWidth=3  IndexOptions=Index vector (dialog),Select all  Indices=[2],1  OutputSizes=1,1
  Selector3 : Selector  NumberOfDimensions=2  InputPortWidth=3  IndexOptions=Index vector (dialog),Select all  Indices=[3],1  OutputSizes=1,1
  Selector4 : Selector  NumberOfDimensions=2  InputPortWidth=3  IndexOptions=Select all,Index vector (dialog)  Indices=[1],2  OutputSizes=1,1
  Selector5 : Selector  NumberOfDimensions=2  InputPortWidth=3  IndexOptions=Select all,Index vector (dialog)  Indices=[1],3  OutputSizes=1,1
  Selector6 : Selector  NumberOfDimensions=2  InputPortWidth=3  IndexOptions=Select all,Index vector (dialog)  Indices=[1],4  OutputSizes=1,1
  Selector7 : Selector  NumberOfDimensions=2  InputPortWidth=3  IndexOptions=Select all,Index vector (dialog)  Indices=[1],1  OutputSizes=1,1
  Sum of Elements : Sum  Inputs=+
  Sum of Elements1 : Sum  Inputs=+
  Sum of Elements2 : Sum  Inputs=+
  Vector Concatenate : Concatenate  NumInputs=3
  Vector Concatenate2 : Concatenate  NumInputs=4
  Fs : Outport  VectorParamsAs1DForOutWhenUnconnected=off
  FVehB : Outport  Port=2  VectorParamsAs1DForOutWhenUnconnected=off
  FxW : Outport  Port=3  VectorParamsAs1DForOutWhenUnconnected=off
  FyW : Outport  Port=4  VectorParamsAs1DForOutWhenUnconnected=off
  FzW : Outport  Port=5  VectorParamsAs1DForOutWhenUnconnected=off
  wires:
  F/1 -> Reshape/1
  Sum of Elements/1 -> Vector Concatenate/1
  Sum of Elements1/1 -> Vector Concatenate/2
  Sum of Elements2/1 -> Vector Concatenate/3
  Vector Concatenate/1 -> FVehB/1
  Selector1/1 -> Reshape1/1
  Selector2/1 -> Reshape2/1
  Selector3/1 -> Reshape3/1
  Vector Concatenate2/1 -> Fs/1
  Selector4/1 -> Vector Concatenate2/2
  Selector7/1 -> Vector Concatenate2/1
  Selector5/1 -> Vector Concatenate2/3
  Reshape/1 -> Selector3/1, Selector2/1, Selector1/1, Selector6/1, Selector5/1, Selector4/1, Selector7/1
  Selector6/1 -> Vector Concatenate2/4
  Reshape1/1 -> FxW/1, Sum of Elements/1
  Reshape2/1 -> FyW/1, Sum of Elements1/1
  Reshape3/1 -> FzW/1, Sum of Elements2/1

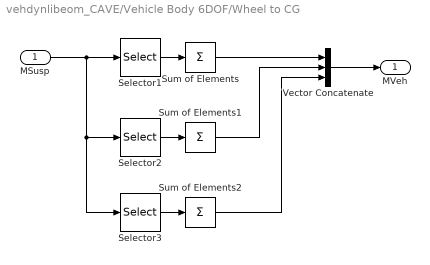
== system vehdynlibeom_CAVE/Vehicle Body 6DOF/Wheel to CG ==
  MSusp : Inport
  Selector1 : Selector  NumberOfDimensions=2  InputPortWidth=3  IndexOptions=Index vector (dialog),Select all  Indices=[1],1  OutputSizes=1,1
  Selector2 : Selector  NumberOfDimensions=2  InputPortWidth=3  IndexOptions=Index vector (dialog),Select all  Indices=[2],1  OutputSizes=1,1
  Selector3 : Selector  NumberOfDimensions=2  InputPortWidth=3  IndexOptions=Index vector (dialog),Select all  Indices=[3],1  OutputSizes=1,1
  Sum of Elements : Sum  Inputs=+
  Sum of Elements1 : Sum  Inputs=+
  Sum of Elements2 : Sum  Inputs=+
  Vector Concatenate : Concatenate  NumInputs=3
  MVeh : Outport  VectorParamsAs1DForOutWhenUnconnected=off
  wires:
  Sum of Elements/1 -> Vector Concatenate/1
  Sum of Elements1/1 -> Vector Concatenate/2
  Sum of Elements2/1 -> Vector Concatenate/3
  Vector Concatenate/1 -> MVeh/1
  MSusp/1 -> Selector3/1, Selector2/1, Selector1/1
  Selector2/1 -> Sum of Elements1/1
  Selector1/1 -> Sum of Elements/1
  Selector3/1 -> Sum of Elements2/1

== system vehdynlibeom_CAVE/Vehicle Body 6DOF/Signal Routing/Hard Point Coordinate Transform Front Left ==
  InertFrmCg : Inport
  BdyFrmCg : Inport  Port=2
  HPbar : Inport  Port=3
  Hard Point Coordinate Transform External Displacement : autolibsharedcommon/Hard Point Coordinate Transform External Displacement  aMode=aMode
      settings: SourceProductName=Powertrain Blockset  SourceProductBaseCode=PW
  Selector1 : Selector  NumberOfDimensions=2  InputPortWidth=3  IndexOptions=Select all,Index vector (dialog)  Indices=[1],[1]  OutputSizes=1,1
  Inert : Outport  VectorParamsAs1DForOutWhenUnconnected=off
  Body : Outport  Port=2  VectorParamsAs1DForOutWhenUnconnected=off
  wires:
  InertFrmCg/1 -> Hard Point Coordinate Transform External Displacement/1
  Hard Point Coordinate Transform External Displacement/2 -> Body/1
  Selector1/1 -> Hard Point Coordinate Transform External Displacement/3
  BdyFrmCg/1 -> Hard Point Coordinate Transform External Displacement/2
  Hard Point Coordinate Transform External Displacement/1 -> Inert/1
  HPbar/1 -> Selector1/1

== system vehdynlibeom_CAVE/Vehicle Body 6DOF/Signal Routing/Hard Point Coordinate Transform Front Right ==
  InertFrmCg : Inport
  BdyFrmCg : Inport  Port=2
  HPbar : Inport  Port=3
  Hard Point Coordinate Transform External Displacement : autolibsharedcommon/Hard Point Coordinate Transform External Displacement  aMode=aMode
      settings: SourceProductName=Powertrain Blockset  SourceProductBaseCode=PW
  Selector1 : Selector  NumberOfDimensions=2  InputPortWidth=3  IndexOptions=Select all,Index vector (dialog)  Indices=[1],[2]  OutputSizes=1,1
  Inert : Outport  VectorParamsAs1DForOutWhenUnconnected=off
  Body : Outport  Port=2  VectorParamsAs1DForOutWhenUnconnected=off
  wires:
  Hard Point Coordinate Transform External Displacement/1 -> Inert/1
  BdyFrmCg/1 -> Hard Point Coordinate Transform External Displacement/2
  Hard Point Coordinate Transform External Displacement/2 -> Body/1
  InertFrmCg/1 -> Hard Point Coordinate Transform External Displacement/1
  HPbar/1 -> Selector1/1
  Selector1/1 -> Hard Point Coordinate Transform External Displacement/3

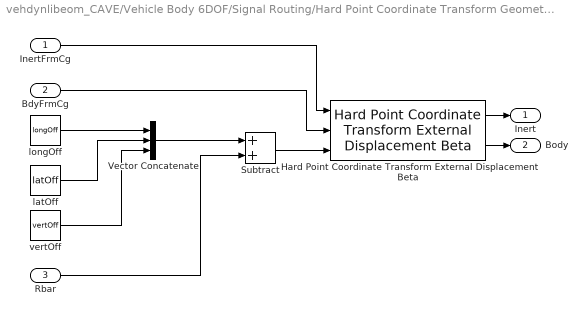
== system vehdynlibeom_CAVE/Vehicle Body 6DOF/Signal Routing/Hard Point Coordinate Transform Geometric ==
  InertFrmCg : Inport
  BdyFrmCg : Inport  Port=2
  Rbar : Inport  Port=3
  Hard Point Coordinate Transform External Displacement Beta : autolibsharedcommon/Hard Point Coordinate Transform External Displacement Beta  xdot_tol=xdot_tol  aMode=aMode
      settings: SourceProductName=Powertrain Blockset  SourceProductBaseCode=PW
  Subtract : Sum
  Vector Concatenate : Concatenate  NumInputs=3
  latOff : Constant  Value=latOff
  longOff : Constant  Value=longOff
  "vertOff " : Constant  Value=vertOff
  Inert : Outport  VectorParamsAs1DForOutWhenUnconnected=off
  Body : Outport  Port=2  VectorParamsAs1DForOutWhenUnconnected=off
  wires:
  InertFrmCg/1 -> Hard Point Coordinate Transform External Displacement Beta/1
  Hard Point Coordinate Transform External Displacement Beta/2 -> Body/1
  Vector Concatenate/1 -> Subtract/1
  BdyFrmCg/1 -> Hard Point Coordinate Transform External Displacement Beta/2
  Hard Point Coordinate Transform External Displacement Beta/1 -> Inert/1
  "vertOff "/1 -> Vector Concatenate/3
  longOff/1 -> Vector Concatenate/1
  latOff/1 -> Vector Concatenate/2
  Rbar/1 -> Subtract/2
  Subtract/1 -> Hard Point Coordinate Transform External Displacement Beta/3

== system vehdynlibeom_CAVE/Vehicle Body 6DOF/Signal Routing/Hard Point Coordinate Transform Rear Left ==
  InertFrmCg : Inport
  BdyFrmCg : Inport  Port=2
  HPbar : Inport  Port=3
  Hard Point Coordinate Transform External Displacement : autolibsharedcommon/Hard Point Coordinate Transform External Displacement  aMode=aMode
      settings: SourceProductName=Powertrain Blockset  SourceProductBaseCode=PW
  Selector1 : Selector  NumberOfDimensions=2  InputPortWidth=3  IndexOptions=Select all,Index vector (dialog)  Indices=[1],[3]  OutputSizes=1,1
  Inert : Outport  VectorParamsAs1DForOutWhenUnconnected=off
  Body : Outport  Port=2  VectorParamsAs1DForOutWhenUnconnected=off
  wires:
  InertFrmCg/1 -> Hard Point Coordinate Transform External Displacement/1
  Hard Point Coordinate Transform External Displacement/2 -> Body/1
  BdyFrmCg/1 -> Hard Point Coordinate Transform External Displacement/2
  Hard Point Coordinate Transform External Displacement/1 -> Inert/1
  HPbar/1 -> Selector1/1
  Selector1/1 -> Hard Point Coordinate Transform External Displacement/3

== system vehdynlibeom_CAVE/Vehicle Body 6DOF/Signal Routing/Hard Point Coordinate Transform Rear Right ==
  InertFrmCg : Inport
  BdyFrmCg : Inport  Port=2
  HPbar : Inport  Port=3
  Hard Point Coordinate Transform External Displacement : autolibsharedcommon/Hard Point Coordinate Transform External Displacement  aMode=aMode
      settings: SourceProductName=Powertrain Blockset  SourceProductBaseCode=PW
  Selector1 : Selector  NumberOfDimensions=2  InputPortWidth=3  IndexOptions=Select all,Index vector (dialog)  Indices=[1],[4]  OutputSizes=1,1
  Inert : Outport  VectorParamsAs1DForOutWhenUnconnected=off
  Body : Outport  Port=2  VectorParamsAs1DForOutWhenUnconnected=off
  wires:
  Hard Point Coordinate Transform External Displacement/1 -> Inert/1
  BdyFrmCg/1 -> Hard Point Coordinate Transform External Displacement/2
  Hard Point Coordinate Transform External Displacement/2 -> Body/1
  InertFrmCg/1 -> Hard Point Coordinate Transform External Displacement/1
  HPbar/1 -> Selector1/1
  Selector1/1 -> Hard Point Coordinate Transform External Displacement/3

== system vehdynlibeom_CAVE/Vehicle Body 6DOF/SignalCollection/Angle Wrap ==
  "u " : Inport
  None : Subsystem  VariantControl=None
  Unwrap : autolibutils/Unwrap  VariantControl=Unwrap  aMode=aMode
      settings: SourceProductName=Powertrain Blockset  SourceProductBaseCode=PW
  " y" : Outport  VectorParamsAs1DForOutWhenUnconnected=off

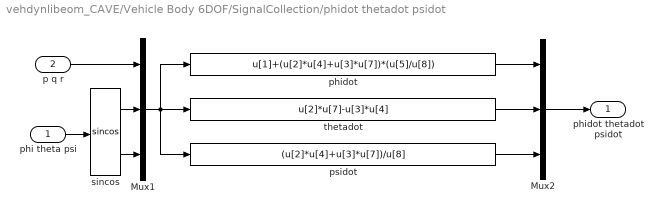
== system vehdynlibeom_CAVE/Vehicle Body 6DOF/SignalCollection/phidot thetadot psidot ==
  phi theta psi : Inport
  p q r : Inport  Port=2
  Mux1 : Mux  Inputs=[3 3 3]
  Mux2 : Mux  Inputs=3
  phidot : Fcn  Expr=u[1]+(u[2]*u[4]+u[3]*u[7])*(u[5]/u[8])
  psidot : Fcn  Expr=(u[2]*u[4]+u[3]*u[7])/u[8]
  sincos : Trigonometry  Operator=sincos
  thetadot : Fcn  Expr=u[2]*u[7]-u[3]*u[4]
  phidot thetadot psidot : Outport  InitialOutput=0  VectorParamsAs1DForOutWhenUnconnected=off
  wires:
  Mux1/1 -> psidot/1, phidot/1, thetadot/1
  p q r/1 -> Mux1/1
  phi theta psi/1 -> sincos/1
  psidot/1 -> Mux2/3
  thetadot/1 -> Mux2/2
  phidot/1 -> Mux2/1
  Mux2/1 -> phidot thetadot psidot/1
  sincos/1 -> Mux1/2
  sincos/2 -> Mux1/3

== system vehdynlibeom_CAVE/Vehicle Body 6DOF/SignalCollection/Angle Wrap/None ==
  u : Inport
  y : Outport  VectorParamsAs1DForOutWhenUnconnected=off
  wires:
  u/1 -> y/1

== matlab function vehdynlibeom_CAVE/Vehicle Body 6DOF/vehdyncginert ==
  data: m parameter size=1; Mbar output size=1; z1m parameter size=1; z2m parameter size=1; z3m parameter size=1; z4m parameter size=1; z5m parameter size=1; z6m parameter size=1; z7m parameter size=1; z1R parameter size=[1,3]; z2R parameter size=[1,3]; z3R parameter size=[1,3]; z4R parameter size=[1,3]; z5R parameter size=[1,3]; z6R parameter size=[1,3]; Iveh parameter size=[3,3]; z1I parameter size=[3,3]; z2I parameter size=[3,3]; z3I parameter size=[3,3]; z4I parameter size=[3,3]; z5I parameter size=[3,3]; z6I parameter size=[3,3]; z7I parameter size=[3,3]; Ibar output size=[3,3]; Rbar output; z7R parameter size=[1,3]; Xbar output; Wbar output; a parameter size=1; b parameter size=1; h parameter size=1; w parameter size=2; d parameter; HPbar output size=[3,4]
function [Mbar,Ibar,Rbar,Xbar,Wbar,HPbar] = inert(m, z1m, z2m, z3m, z4m, z5m, z6m, z7m,z1R, z2R, z3R, z4R, z5R, z6R, Iveh, z1I, z2I, z3I, z4I, z5I, z6I, z7I, z7R, a, b, h, w, d)%#codegen
coder.allowpcode('plain')
[Rbar,Mbar,Ibar,Xbar,Wbar,HPbar]= vehdyncginerthp(m, z1m, z2m, z3m, z4m, z5m, z6m, z7m,z1R, z2R, z3R, z4R, z5R, z6R, Iveh, z1I, z2I, z3I, z4I, z5I, z6I, z7I, z7R, a, b, h, w, d);
end
